simulink model "therac_statechart_sldv_d"  (Simulink 8.7)
settings: Solver=FixedStepDiscrete  StartTime=0.0  StopTime=30  FixedStep=1  RelTol=1e-3
libraries: sldvlib x4
settings DataIOCC: LimitDataPoints=off  SaveFormat=Dataset
settings DebuggingCC: UnderspecifiedInitializationDetection=Simplified  MergeDetectMultiDrivingBlocksExec=error
settings HardwareCC: ProdBitPerPointer=64  ProdLargestAtomicFloat=Float  ProdIntDivRoundTo=Zero  ProdEndianess=LittleEndian  ProdWordSize=64  ProdHWDeviceType=Intel->x86-64 (Windows64)
settings ModelReferenceCC: PropagateSignalLabelsOutOfModel=on
settings ConfigComp: CovModelRefEnable=off

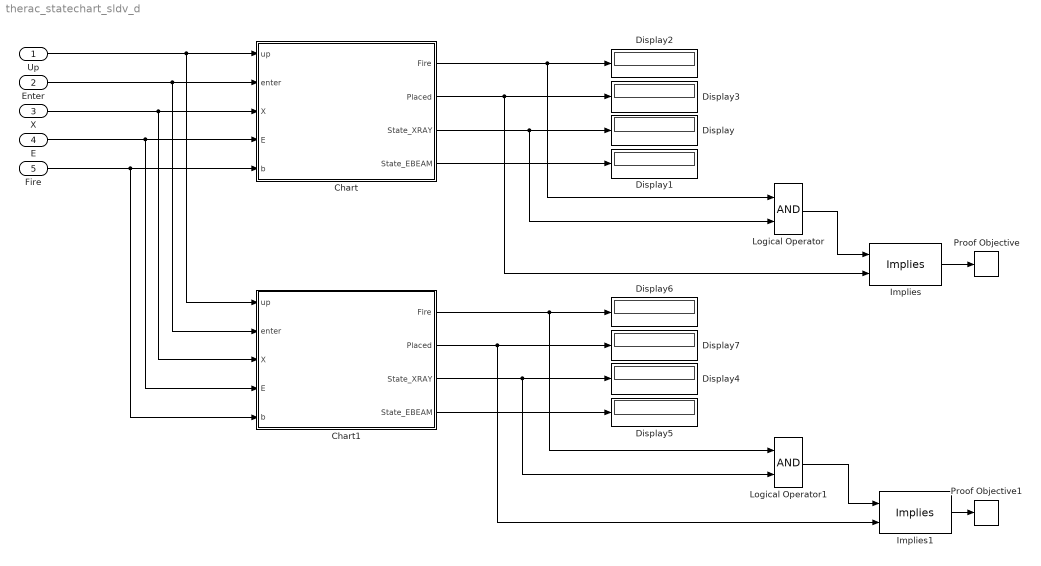
== system therac_statechart_sldv_d ==
  Up : Inport  OutDataTypeStr=boolean
  Enter : Inport  Port=2  OutDataTypeStr=boolean
  X : Inport  Port=3  OutDataTypeStr=boolean
  E : Inport  Port=4  OutDataTypeStr=boolean
  Fire : Inport  Port=5  OutDataTypeStr=boolean
  Chart : Stateflow chart  TreatAsAtomicUnit=on
  Chart1 : Stateflow chart  TreatAsAtomicUnit=on
  Display{,1..7} (8 alike) : Display
  Implies : sldvlib/Verification Utilities/Implies
  Implies1 : sldvlib/Verification Utilities/Implies
  Logical Operator : Logic  AllPortsSameDT=off  OutDataTypeStr=boolean
  Logical Operator1 : Logic  AllPortsSameDT=off  OutDataTypeStr=boolean
  Proof Objective : sldvlib/Objectives and Constraints/Proof Objective  enabled=on  customAVTBlockType=Proof Objective  intervals=true  dispValues=on  outEnabled=off  enableStopSim=off
      settings: AttributesFormatString=%<intervals>
  Proof Objective1 : sldvlib/Objectives and Constraints/Proof Objective  enabled=on  customAVTBlockType=Proof Objective  intervals=true  dispValues=on  outEnabled=off  enableStopSim=off
      settings: AttributesFormatString=%<intervals>
  wires:
  Chart/1(Fire) -> Logical Operator/1, Display2/1
  Chart/2(Placed) -> Implies/2, Display3/1
  Chart/4(State_EBEAM) -> Display1/1
  Up/1 -> Chart1/1(up), Chart/1(up)
  Enter/1 -> Chart1/2(enter), Chart/2(enter)
  X/1 -> Chart1/3(X), Chart/3(X)
  E/1 -> Chart1/4(E), Chart/4(E)
  Fire/1 -> Chart1/5(b), Chart/5(b)
  Chart/3(State_XRAY) -> Logical Operator/2, Display/1
  Logical Operator/1 -> Implies/1
  Implies/1 -> Proof Objective/1
  Chart1/1(Fire) -> Logical Operator1/1, Display6/1
  Chart1/2(Placed) -> Implies1/2, Display7/1
  Chart1/4(State_EBEAM) -> Display5/1
  Chart1/3(State_XRAY) -> Logical Operator1/2, Display4/1
  Logical Operator1/1 -> Implies1/1
  Implies1/1 -> Proof Objective1/1

== stateflow chart Chart1 ==
  state Interface [parallel]
    settings: executionOrder=1
    state Edit
    state XRay
      state XDataEntry
      state XDataReady
      XDataReady -> XDataEntry [order 1] : [up]
      XDataEntry -> XDataReady [order 2] : [enter]
    state EBeam
      state EDataEntry
      state EDataReady
      EDataEntry -> EDataReady [order 2] : [enter]
      EDataReady -> EDataEntry [order 1] : [up]
    state Treatment_Administered
    (default) -> Edit
    Treatment_Administered -> Edit : [enter]
    EDataEntry -> Edit [order 1] : [up]
    XDataEntry -> Edit [order 1] : [up]
    Edit -> XDataEntry [order 1] : [X]
        | /{BeamLevel.SELECT_X,
        | Spreader.SELECT_X}
    Edit -> EDataEntry [order 2] : [E]
        | /{BeamLevel.SELECT_E,
        | Spreader.SELECT_E}
    EDataReady -> Treatment_Administered [order 2] : [b]/{BeamFire.FIRE}
    XDataReady -> Treatment_Administered [order 2] : [b && in(Spreader.InPlace)]/{BeamFire.FIRE}
  state BeamLevel [parallel]
    settings: executionOrder=2
    state Neither
      entry: State_XRAY=false;
      State_EBEAM=false;
    state X
      entry: State_XRAY=true;
      State_EBEAM=false;
      state XSet
      state XtoE
      (default) -> XSet
      XSet -> XtoE : SELECT_E
    state E
      entry: State_XRAY=false;
      State_EBEAM=true;
      state ESet
      state EtoX
      (default) -> ESet
      ESet -> EtoX : SELECT_X
    (default) -> Neither
    X -> Neither : RESET
    E -> Neither : RESET
    Neither -> X [order 1] : SELECT_X
    Neither -> E [order 2] : SELECT_E
    XtoE -> E : after(1,tick)
    EtoX -> X : after(1,tick)
  state Spreader [parallel]
    settings: executionOrder=3
    state OutOfPlace
      entry:
      Placed=false;
    state InPlace
      entry:
      Placed=true;
    state MovingInPlace
    state MovingOut
    InPlace -> MovingOut : SELECT_E
    MovingOut -> OutOfPlace [order 1] : after(8,tick)
    (default) -> InPlace
    MovingOut -> MovingInPlace [order 2] : SELECT_X
    MovingInPlace -> MovingOut [order 1] : SELECT_E
    OutOfPlace -> MovingInPlace : SELECT_X
    MovingInPlace -> InPlace [order 2] : after(8,tick)
  state BeamFire [parallel]
    settings: executionOrder=4
    state Waiting
      entry: Fire=false;
    state Fired
      entry: Fire=true;
    Fired -> Waiting : after(1,tick)/{BeamLevel.RESET}
    (default) -> Waiting
    Waiting -> Fired : FIRE
  data: up input boolean; enter input boolean; X input boolean; E input boolean; b input boolean; Fire output boolean; Placed output boolean; State_XRAY output boolean; State_EBEAM output boolean
  events: RESET local FUNCTION_CALL_EVENT; SELECT_X local FUNCTION_CALL_EVENT; SELECT_E local FUNCTION_CALL_EVENT; SELECT_X local FUNCTION_CALL_EVENT; SELECT_E local FUNCTION_CALL_EVENT; FIRE local FUNCTION_CALL_EVENT

== stateflow chart Chart ==
  state Interface [parallel]
    settings: executionOrder=1
    state Edit
    state XRay
      state XDataEntry
      state XDataReady
      XDataReady -> XDataEntry [order 1] : [up]
      XDataEntry -> XDataReady [order 2] : [enter]
    state EBeam
      state EDataEntry
      state EDataReady
      EDataEntry -> EDataReady [order 2] : [enter]
      EDataReady -> EDataEntry [order 1] : [up]
    state Treatment_Administered
    (default) -> Edit
    Treatment_Administered -> Edit : [enter]
    EDataEntry -> Edit [order 1] : [up]
    XDataEntry -> Edit [order 1] : [up]
    Edit -> XDataEntry [order 1] : [X]
        | /{BeamLevel.SELECT_X,
        | Spreader.SELECT_X}
    Edit -> EDataEntry [order 2] : [E]
        | /{BeamLevel.SELECT_E,
        | Spreader.SELECT_E}
    EDataReady -> Treatment_Administered [order 2] : [b]/{BeamFire.FIRE}
    XDataReady -> Treatment_Administered [order 2] : [b]/{BeamFire.FIRE}
  state BeamLevel [parallel]
    settings: executionOrder=2
    state Neither
      entry: State_XRAY=false;
      State_EBEAM=false;
    state X
      entry: State_XRAY=true;
      State_EBEAM=false;
      state XSet
      state XtoE
      (default) -> XSet
      XSet -> XtoE : SELECT_E
    state E
      entry: State_XRAY=false;
      State_EBEAM=true;
      state ESet
      state EtoX
      (default) -> ESet
      ESet -> EtoX : SELECT_X
    (default) -> Neither
    X -> Neither : RESET
    E -> Neither : RESET
    Neither -> E [order 2] : SELECT_E
    Neither -> X [order 1] : SELECT_X
    XtoE -> E : after(1,tick)
    EtoX -> X : after(1,tick)
  state Spreader [parallel]
    settings: executionOrder=3
    state OutOfPlace
      entry:
      Placed=false;
    state InPlace
      entry:
      Placed=true;
    state MovingInPlace
    state MovingOut
    InPlace -> MovingOut : SELECT_E
    MovingOut -> OutOfPlace [order 1] : after(8,tick)
    (default) -> InPlace
    MovingOut -> MovingInPlace [order 2] : SELECT_X
    MovingInPlace -> MovingOut [order 1] : SELECT_E
    OutOfPlace -> MovingInPlace : SELECT_X
    MovingInPlace -> InPlace [order 2] : after(8,tick)
  state BeamFire [parallel]
    settings: executionOrder=4
    state Waiting
      entry: Fire=false;
    state Fired
      entry: Fire=true;
    Fired -> Waiting : after(1,tick)/{BeamLevel.RESET}
    (default) -> Waiting
    Waiting -> Fired : FIRE
  data: up input boolean; enter input boolean; X input boolean; E input boolean; b input boolean; Fire output boolean; Placed output boolean; State_XRAY output boolean; State_EBEAM output boolean
  events: RESET local FUNCTION_CALL_EVENT; SELECT_X local FUNCTION_CALL_EVENT; SELECT_E local FUNCTION_CALL_EVENT; SELECT_X local FUNCTION_CALL_EVENT; SELECT_E local FUNCTION_CALL_EVENT; FIRE local FUNCTION_CALL_EVENT
